simulink model "TCS_Implementation_Controllers"  (R2023b)
settings: Solver=FixedStepDiscrete  StartTime=0.0  StopTime=inf  FixedStep=0.005  RelTol=1e-3  EnableMultiTasking=on
undefined symbols (not defined in the file): bits, DiscIntNeverNeededParam
libraries: stm32f4xxblockslib x19, simulink x17, stm32blockslib x11, dspstat3 x4, embeddedblockslib x3, eeGeneralControl x2, slpidlib x2, mspfiltlib x1
(part 1 of 2)
settings Model: Creator=ADMIN  LastModifiedBy=ADMIN
settings OptimizationCC: EnhancedBackFolding=on  PassReuseOutputArgsAs=Individual arguments  ZeroExternalMemoryAtStartup=off  ZeroInternalMemoryAtStartup=off  MaxStackSize=64  OptimizeBlockOrder=speed  DifferentSizesBufferReuse=on  OptimizationCustomize=off  EfficientTunableParamExpr=on
settings DebuggingCC: MultiTaskDSMMsg=none  TasksWithSamePriorityMsg=none  ParameterPrecisionLossMsg=none  ParameterTunabilityLossMsg=error
settings HardwareCC: ProdBitPerPointer=32  ProdBitPerSizeT=32  ProdBitPerPtrDiffT=32  ProdLargestAtomicInteger=Long  ProdLargestAtomicFloat=Double  ProdWordSize=32  ProdLongLongMode=on  ProdHWDeviceType=ARM Compatible->ARM Cortex
settings SFSimCC: MATLABDynamicMemAlloc=off
settings RTWCC: Description=Embedded Coder  SystemTargetFile=ert.tlc  HardwareBoard=STM32F4xx Based  TemplateMakefile=ert_default_tmf  Toolchain=GNU Tools for ARM Embedded Processors
settings CodeAppCC: ForceParamTrailComments=on  IgnoreCustomStorageClasses=off  OperatorAnnotations=on  SimulinkDataObjDesc=on  SFDataObjDesc=on  InsertBlockDesc=on
settings ERTTargetCC: CodeReplacementLibrary=ARM Cortex-M  ExtModeTransport=3  ExtModeStaticAlloc=on  ExtModeStaticAllocSize=2048  ExtModeMexFile=ext_xcp  ExtModeIntrfLevel=Level2 - Open

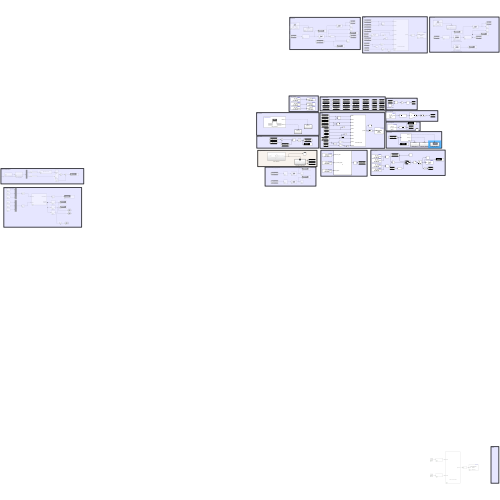
[thumbnail: Simulink's stored preview of the top-level diagram]
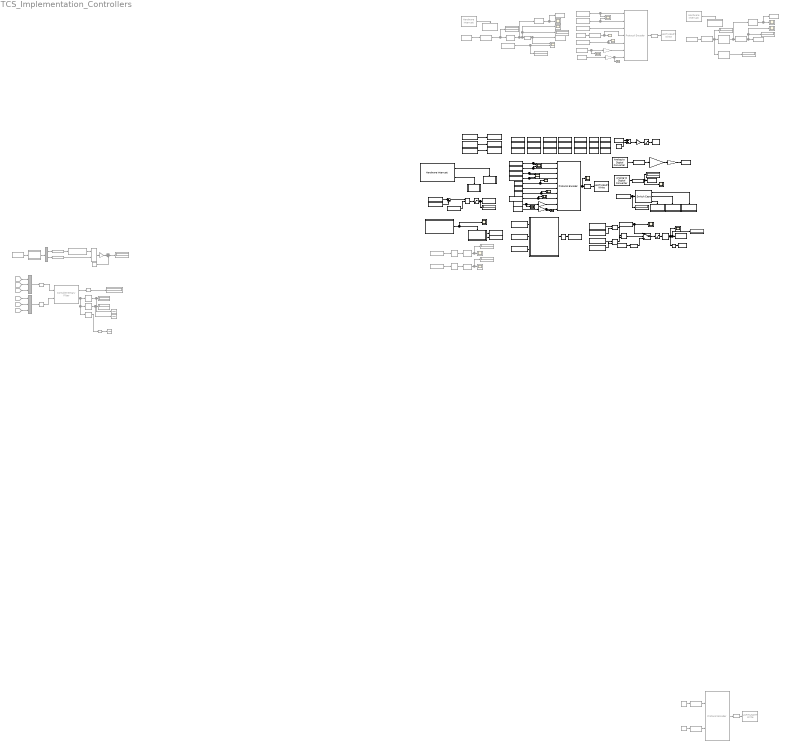
== system TCS_Implementation_Controllers ==
  note: ACC_Calculation_By_System
  note: Torque Sense
  note: Slip_Ratio
  note: WS_Front
  note: Global Variables
  note: Complemetary Filter
  note: WS_Timer
  note: UART
  note: OutPut_DAC
  note: Condition Controller
  note: Controllers
  note: WS_Rear
  note: Throttle Signals
  note: UART
  note: Read Temperature
  note: Signal_LEDs
  note: UART
  note: Current Sense
  note: ACC_Calculation
  AND : Logic  IconShape=distinctive  AllPortsSameDT=off  OutDataTypeStr=boolean
  AND1 : Logic  IconShape=distinctive  AllPortsSameDT=off  OutDataTypeStr=boolean
  Analog to Digital Converter : stm32f4xxblockslib/Analog to Digital Converter  ADCModule=ADC2  ConversionGroup=Regular  TriggerMode=Trigger and read  NumberOfConversions=1  EnableBufferConv=off  BufferLength=1  OutputStatus=off  SampleTime=-1  EnableSimPort=off
  Analog to Digital Converter1 : stm32f4xxblockslib/Analog to Digital Converter  ADCModule=ADC1  ConversionGroup=Regular  TriggerMode=Trigger and read  NumberOfConversions=1  EnableBufferConv=off  BufferLength=1  OutputStatus=off  SampleTime=-1  EnableSimPort=off
  Bitwise Operator7 : simulink/Logic and Bit Operations/Bitwise Operator  Commented=on  logicop=OR  UseBitMask=off  NumInputPorts=2  BitMask=bin2dec('11011001')  BitMaskRealWorld=Stored Integer
  Calculate Acceleration : Subsystem
  Calibrated value : Constant  Value=5  OutDataTypeStr=single
  Complementary Filter : mspfiltlib/Complementary Filter  Commented=on  DispRefFrame=ENU  OrientationFormat=quaternion  AccelerometerGain=0.05  HasMagnetometer=off  MagnetometerGain=0.01  SimulateUsing=Interpreted execution
  Configuration for Accelerometer1 : Constant  Commented=on  Value=hex2dec('0')  OutDataTypeStr=uint8
  Constant1 : Constant  Commented=on  Value=36.35
  Data Store Memory : DataStoreMemory  DataStoreName=WS1_Pulse  WriteAfterWriteMsg=warning  ShowAdditionalParam=off  OutDataTypeStr=uint32
  Data Store Memory1 : DataStoreMemory  DataStoreName=WS2_Pulse  WriteAfterWriteMsg=warning  ShowAdditionalParam=off  OutDataTypeStr=uint32
  Data Store Memory10 : DataStoreMemory  DataStoreName=WS1_ACC_Timer  WriteAfterWriteMsg=warning  ShowAdditionalParam=off  OutDataTypeStr=single
  Data Store Memory11 : DataStoreMemory  DataStoreName=WS2_ACC_Timer  WriteAfterWriteMsg=warning  ShowAdditionalParam=off  OutDataTypeStr=single
  Data Store Memory12 : DataStoreMemory  DataStoreName=WS1_Speed_Timer  WriteAfterWriteMsg=warning  ShowAdditionalParam=off  OutDataTypeStr=single
  Data Store Memory13 : DataStoreMemory  DataStoreName=WS2_Speed_Timer  WriteAfterWriteMsg=warning  ShowAdditionalParam=off  OutDataTypeStr=single
  Data Store Memory14 : DataStoreMemory  DataStoreName=Slip_Ratio  WriteAfterWriteMsg=warning  ShowAdditionalParam=off  OutDataTypeStr=single
  Data Store Memory15 : DataStoreMemory  DataStoreName=DAC_Out  WriteAfterWriteMsg=warning  InitialValue=900  ShowAdditionalParam=off  OutDataTypeStr=uint16
  Data Store Memory16 : DataStoreMemory  DataStoreName=Controller_State  WriteAfterWriteMsg=warning  InitialValue=1100  ShowAdditionalParam=off  OutDataTypeStr=uint16
  Data Store Memory17 : DataStoreMemory  DataStoreName=Roll_Angle  WriteAfterWriteMsg=warning  ShowAdditionalParam=off  OutDataTypeStr=single
  Data Store Memory18 : DataStoreMemory  DataStoreName=Pitch_Angle  WriteAfterWriteMsg=warning  ShowAdditionalParam=off  OutDataTypeStr=single
  Data Store Memory19 : DataStoreMemory  DataStoreName=Yaw_Angle  WriteAfterWriteMsg=warning  ShowAdditionalParam=off  OutDataTypeStr=single
  Data Store Memory2 : DataStoreMemory  DataStoreName=WS1_Speed  WriteAfterWriteMsg=warning  ShowAdditionalParam=off  OutDataTypeStr=single
  Data Store Memory20 : DataStoreMemory  DataStoreName=Yaw_Rate  WriteAfterWriteMsg=warning  ShowAdditionalParam=off  OutDataTypeStr=single
  Data Store Memory3 : DataStoreMemory  DataStoreName=WS2_Speed  WriteAfterWriteMsg=warning  ShowAdditionalParam=off  OutDataTypeStr=single
  Data Store Memory4 : DataStoreMemory  DataStoreName=Throttle_In  WriteAfterWriteMsg=warning  ShowAdditionalParam=off  OutDataTypeStr=single
  Data Store Memory5 : DataStoreMemory  DataStoreName=Current  WriteAfterWriteMsg=warning  ShowAdditionalParam=off  OutDataTypeStr=single
  Data Store Memory6 : DataStoreMemory  DataStoreName=Throttle_Out  WriteAfterWriteMsg=warning  ShowAdditionalParam=off  OutDataTypeStr=single
  Data Store Memory7 : DataStoreMemory  DataStoreName=Torque  WriteAfterWriteMsg=warning  ShowAdditionalParam=off  OutDataTypeStr=single
  Data Store Memory8 : DataStoreMemory  DataStoreName=WS1_ACC  WriteAfterWriteMsg=warning  ShowAdditionalParam=off  OutDataTypeStr=single
  Data Store Memory9 : DataStoreMemory  DataStoreName=WS2_ACC  WriteAfterWriteMsg=warning  ShowAdditionalParam=off  OutDataTypeStr=single
  Data Store Read : DataStoreRead  Commented=on  DataStoreName=WS2_Pulse  IndexOptions=Index vector (dialog)  Indices=1  OutputSizes=1
  Data Store Read1 : DataStoreRead  DataStoreName=WS1_ACC_Timer  IndexOptions=Index vector (dialog)  Indices=1  OutputSizes=1
  Data Store Read10 : DataStoreRead  Commented=on  DataStoreName=WS2_Speed_Timer  IndexOptions=Index vector (dialog)  Indices=1  OutputSizes=1
  Data Store Read11 : DataStoreRead  DataStoreName=WS2_Speed_Timer  IndexOptions=Index vector (dialog)  Indices=1  OutputSizes=1
  Data Store Read12 : DataStoreRead  DataStoreName=Slip_Ratio  IndexOptions=Index vector (dialog)  Indices=1  OutputSizes=1
  Data Store Read13 : DataStoreRead  DataStoreName=Throttle_In  IndexOptions=Index vector (dialog)  Indices=1  OutputSizes=1
  Data Store Read14 : DataStoreRead  DataStoreName=Controller_State  IndexOptions=Index vector (dialog)  Indices=1  OutputSizes=1
  Data Store Read15 : DataStoreRead  DataStoreName=DAC_Out  IndexOptions=Index vector (dialog)  Indices=1  OutputSizes=1
  Data Store Read16 : DataStoreRead  DataStoreName=Current  IndexOptions=Index vector (dialog)  Indices=1  OutputSizes=1
  Data Store Read17 : DataStoreRead  Commented=on  DataStoreName=Slip_Ratio  IndexOptions=Index vector (dialog)  Indices=1  OutputSizes=1
  Data Store Read18 : DataStoreRead  DataStoreName=WS2_ACC_Timer  IndexOptions=Index vector (dialog)  Indices=1  OutputSizes=1
  Data Store Read19 : DataStoreRead  DataStoreName=Torque  IndexOptions=Index vector (dialog)  Indices=1  OutputSizes=1
  Data Store Read2 : DataStoreRead  DataStoreName=WS1_Speed_Timer  IndexOptions=Index vector (dialog)  Indices=1  OutputSizes=1
  Data Store Read20 : DataStoreRead  DataStoreName=Current  IndexOptions=Index vector (dialog)  Indices=1  OutputSizes=1
  Data Store Read22 : DataStoreRead  DataStoreName=Throttle_In  IndexOptions=Index vector (dialog)  Indices=1  OutputSizes=1
  Data Store Read23 : DataStoreRead  Commented=on  DataStoreName=Throttle_In  IndexOptions=Index vector (dialog)  Indices=1  OutputSizes=1
  Data Store Read24 : DataStoreRead  Commented=on  DataStoreName=Current  IndexOptions=Index vector (dialog)  Indices=1  OutputSizes=1
  Data Store Read25 : DataStoreRead  Commented=on  DataStoreName=WS2_ACC_Timer  IndexOptions=Index vector (dialog)  Indices=1  OutputSizes=1
  Data Store Read26 : DataStoreRead  Commented=on  DataStoreName=WS1_Speed_Timer  IndexOptions=Index vector (dialog)  Indices=1  OutputSizes=1
  Data Store Read27 : DataStoreRead  Commented=on  DataStoreName=WS1_Speed_Timer  IndexOptions=Index vector (dialog)  Indices=1  OutputSizes=1
  Data Store Read28 : DataStoreRead  Commented=on  DataStoreName=WS2_Speed_Timer  IndexOptions=Index vector (dialog)  Indices=1  OutputSizes=1
  Data Store Read29 : DataStoreRead  Commented=on  DataStoreName=WS2_Speed_Timer  IndexOptions=Index vector (dialog)  Indices=1  OutputSizes=1
  Data Store Read3 : DataStoreRead  DataStoreName=WS2_Speed_Timer  IndexOptions=Index vector (dialog)  Indices=1  OutputSizes=1
  Data Store Read31 : DataStoreRead  Commented=on  DataStoreName=Throttle_Out  IndexOptions=Index vector (dialog)  Indices=1  OutputSizes=1
  Data Store Read5 : DataStoreRead  DataStoreName=WS1_Speed_Timer  IndexOptions=Index vector (dialog)  Indices=1  OutputSizes=1
  Data Store Read6 : DataStoreRead  DataStoreName=Torque  IndexOptions=Index vector (dialog)  Indices=1  OutputSizes=1
  Data Store Read7 : DataStoreRead  DataStoreName=Throttle_Out  IndexOptions=Index vector (dialog)  Indices=1  OutputSizes=1
  Data Store Read8 : DataStoreRead  Commented=on  DataStoreName=WS1_Pulse  IndexOptions=Index vector (dialog)  Indices=1  OutputSizes=1
  Data Store Read9 : DataStoreRead  DataStoreName=WS2_Speed_Timer  IndexOptions=Index vector (dialog)  Indices=1  OutputSizes=1
  Data Store Write : DataStoreWrite  DataStoreName=Throttle_In  IndexOptions=Index vector (dialog)  Indices=1  OutputSizes=1
  Data Store Write1 : DataStoreWrite  Commented=on  DataStoreName=WS2_Speed  IndexOptions=Index vector (dialog)  Indices=1  OutputSizes=1
  Data Store Write10 : DataStoreWrite  DataStoreName=Slip_Ratio  IndexOptions=Index vector (dialog)  Indices=1  OutputSizes=1
  Data Store Write11 : DataStoreWrite  DataStoreName=Controller_State  IndexOptions=Index vector (dialog)  Indices=1  OutputSizes=1
  Data Store Write15 : DataStoreWrite  DataStoreName=Torque  IndexOptions=Index vector (dialog)  Indices=1  OutputSizes=1
  Data Store Write2 : DataStoreWrite  DataStoreName=Throttle_Out  IndexOptions=Index vector (dialog)  Indices=1  OutputSizes=1
  Data Store Write3 : DataStoreWrite  DataStoreName=Current  IndexOptions=Index vector (dialog)  Indices=1  OutputSizes=1
  Data Store Write4 : DataStoreWrite  DataStoreName=WS1_ACC_Timer  IndexOptions=Index vector (dialog)  Indices=1  OutputSizes=1
  Data Store Write5 : DataStoreWrite  DataStoreName=WS2_ACC_Timer  IndexOptions=Index vector (dialog)  Indices=1  OutputSizes=1
  Data Store Write6 : DataStoreWrite  Commented=on  DataStoreName=WS2_ACC  IndexOptions=Index vector (dialog)  Indices=1  OutputSizes=1
  Data Store Write7 : DataStoreWrite  Commented=on  DataStoreName=WS1_Speed  IndexOptions=Index vector (dialog)  Indices=1  OutputSizes=1
  Data Store Write8 : DataStoreWrite  Commented=on  DataStoreName=WS1_ACC  IndexOptions=Index vector (dialog)  Indices=1  OutputSizes=1
  Data Type Conversion : DataTypeConversion  Commented=on  OutDataTypeStr=double  SaturateOnIntegerOverflow=off  RndMeth=Floor
  Data Type Conversion1 : DataTypeConversion  OutDataTypeStr=single  SaturateOnIntegerOverflow=off  RndMeth=Floor
  Data Type Conversion10 : DataTypeConversion  OutDataTypeStr=uint16  SaturateOnIntegerOverflow=off  RndMeth=Floor
  Data Type Conversion18 : DataTypeConversion  Commented=on  OutDataTypeStr=int16  SaturateOnIntegerOverflow=off  RndMeth=Floor
  Data Type Conversion19 : DataTypeConversion  Commented=on  OutDataTypeStr=int16  SaturateOnIntegerOverflow=off  RndMeth=Floor
  Data Type Conversion{2..3,6,8} (4 alike) : DataTypeConversion  Commented=on  OutDataTypeStr=single  SaturateOnIntegerOverflow=off  RndMeth=Floor
  Data Type Conversion25 : DataTypeConversion  OutDataTypeStr=single  SaturateOnIntegerOverflow=off  RndMeth=Floor
  Data Type Conversion4 : DataTypeConversion  OutDataTypeStr=single  SaturateOnIntegerOverflow=off  RndMeth=Floor
  Data Type Conversion5 : DataTypeConversion  Commented=on  OutDataTypeStr=double  SaturateOnIntegerOverflow=off  RndMeth=Floor
  Data Type Conversion7 : DataTypeConversion  OutDataTypeStr=uint16  SaturateOnIntegerOverflow=off  RndMeth=Floor
  Demux1 : Demux  Commented=on  Outputs=2
  Digital Port Read{1,4..5,10} (4 alike) : stm32f4xxblockslib/Digital Port Read  PortName=GPIOC  PinNumber=[7]  ReadOperation=on  IOAsArray=on  SampleTime=-1  EnableSimPort=off
  Digital Port Read11 : stm32f4xxblockslib/Digital Port Read  PortName=GPIOA  PinNumber=[12]  ReadOperation=on  IOAsArray=on  SampleTime=-1  EnableSimPort=off
  Digital Port Read2 : stm32f4xxblockslib/Digital Port Read  PortName=GPIOA  PinNumber=[11]  ReadOperation=on  IOAsArray=on  SampleTime=-1  EnableSimPort=off
  Digital Port Read6 : stm32f4xxblockslib/Digital Port Read  PortName=GPIOA  PinNumber=[12]  ReadOperation=on  IOAsArray=on  SampleTime=-1  EnableSimPort=off
  Digital Port Read7 : stm32f4xxblockslib/Digital Port Read  PortName=GPIOA  PinNumber=[11]  ReadOperation=on  IOAsArray=on  SampleTime=-1  EnableSimPort=off
  Digital Port Read8 : stm32f4xxblockslib/Digital Port Read  PortName=GPIOA  PinNumber=[12]  ReadOperation=on  IOAsArray=on  SampleTime=-1  EnableSimPort=off
  Digital Port Read9 : stm32f4xxblockslib/Digital Port Read  PortName=GPIOA  PinNumber=[11]  ReadOperation=on  IOAsArray=on  SampleTime=-1  EnableSimPort=off
  Digital Port Write3 : stm32f4xxblockslib/Digital Port Write  PortName=GPIOC  PinNumber=[6]  ReadOperation=off  IOAsArray=on  EnableSimPort=off
  Digital Port Write4 : stm32f4xxblockslib/Digital Port Write  PortName=GPIOC  PinNumber=[8]  ReadOperation=off  IOAsArray=on  EnableSimPort=off
  Digital Port Write5 : stm32f4xxblockslib/Digital Port Write  PortName=GPIOC  PinNumber=[5]  ReadOperation=off  IOAsArray=on  EnableSimPort=off
  Digital to Analog Converter1 : stm32blockslib/Digital to Analog Converter  DACModule=DAC1  TriggerType=Write only  ChannelGroup=Channel1  waveGenEnable=off  waveType=Noise/Triangular  TriggerEnable=on  stepTriggerEnable=on  resetTriggerEnable=on  TrigConfig=Independent trigger  DataLength=12 bits  DataAlignment=Right alignment  dacEnable=off  OutputStatus=off
      settings: LibrarySourceBlock=stm32f4xxblockslib/Digital to Analog Converter
  Discrete Derivative : simulink/Discrete/Discrete Derivative  Commented=on  gainval=(pi*0.41/50)  ICPrevScaledInput=0.0  OutMin=[]  OutMax=[]  OutDataType=fixdt(1, 16)  OutScaling=2^-10  DoSatur=off
  Discrete Derivative2 : simulink/Discrete/Discrete Derivative  Commented=on  gainval=1  ICPrevScaledInput=0  OutMin=[]  OutMax=[]  OutDataTypeStr=single  OutputDataTypeScalingMode=single  OutDataType=fixdt(1, 16)  OutScaling=2^-10  DoSatur=off
  Discrete Derivative3 : simulink/Discrete/Discrete Derivative  Commented=on  gainval=1  ICPrevScaledInput=0  OutMin=[]  OutMax=[]  OutDataTypeStr=single  OutputDataTypeScalingMode=single  OutDataType=fixdt(1, 16)  OutScaling=2^-10  DoSatur=off
  Discrete Derivative5 : simulink/Discrete/Discrete Derivative  Commented=on  gainval=1  ICPrevScaledInput=0.0  OutMin=[]  OutMax=[]  OutDataType=fixdt(1, 16)  OutScaling=2^-10  DoSatur=off
  Discrete Derivative6 : simulink/Discrete/Discrete Derivative  Commented=on  gainval=1  ICPrevScaledInput=0.0  OutMin=[]  OutMax=[]  OutDataType=fixdt(1, 16)  OutScaling=2^-10  DoSatur=off
  Discrete-Time Integrator4 : DiscreteIntegrator  Commented=on  SampleTime=0.005  ICPrevOutput=DiscIntNeverNeededParam  ICPrevScaledInput=DiscIntNeverNeededParam
  Discrete-Time Integrator5 : DiscreteIntegrator  Commented=on  SampleTime=0.005  ICPrevOutput=DiscIntNeverNeededParam  ICPrevScaledInput=DiscIntNeverNeededParam
  Discrete-Time Integrator6 : DiscreteIntegrator  Commented=on  ICPrevOutput=DiscIntNeverNeededParam  ICPrevScaledInput=DiscIntNeverNeededParam
  Display{,1,5..6,8..12,14,17..18} (12 alike) : Display  Commented=on
  Display{2..4,7} (4 alike) : Display
  Divide1 : Product  Inputs=*/
  Filtered Derivative (Discrete or Continuous)1 : eeGeneralControl/Filtered Derivative (Discrete or Continuous)  Commented=on  K=pi*0.4668/50  T=0.1  B=90  A=0  minRatio=5  init_option=Inherited from block input  x0=0  Ts=-1
      settings: LibrarySourceBlock=|
      | ee_sl_lib/General Control/Filtered Derivative
      | (Discrete or Continuous)
  Filtered Derivative (Discrete or Continuous)2 : eeGeneralControl/Filtered Derivative (Discrete or Continuous)  Commented=on  K=60/50  T=0.1  B=2000  A=0  minRatio=5  init_option=Inherited from block input  x0=0  Ts=-1
      settings: LibrarySourceBlock=|
      | ee_sl_lib/General Control/Filtered Derivative
      | (Discrete or Continuous)
  From10 : From  Commented=on  GotoTag=Gryro_Z
  From11 : From  Commented=on  GotoTag=Gryro_Y
  From12 : From  Commented=on  GotoTag=Gryro_X
  From13 : From  Commented=on  GotoTag=Gryro_Z
  From14 : From  Commented=on  GotoTag=Acc_Y
  From15 : From  Commented=on  GotoTag=Acc_X
  Function-Call Subsystem : Subsystem  Commented=on  TreatAsAtomicUnit=on
  Function-Call Subsystem1 : Subsystem  Commented=on  TreatAsAtomicUnit=on
  Function-Call Subsystem2 : Subsystem  TreatAsAtomicUnit=on
  Function-Call Subsystem3 : Subsystem  TreatAsAtomicUnit=on
  Gain : Gain  Gain=(3300/4096)/40  OutDataTypeStr=single
  Gain10 : Gain  Commented=on  Gain=1/340  OutDataTypeStr=single
  Gain11 : Gain  Gain=1.5  OutDataTypeStr=single
  Gain12 : Gain  Commented=on  Gain=3.3/4096  OutDataTypeStr=single
  Gain13 : Gain  Commented=on  Gain=3.3/4096  OutDataTypeStr=single
  Gain2 : Gain  Gain=1/0.75  OutDataTypeStr=single
  Gain3 : Gain  Gain=3.3/4096  OutDataTypeStr=single
  Gain4 : Gain  Gain=3.3/4096  OutDataTypeStr=single
  Get Temp data : Subsystem  Commented=on
  Hardware Interrupt : stm32f4xxblockslib/Hardware Interrupt  Commented=on  ISRGroup=External interrupts (EXTI)  ISRName=EXTI15_10_IRQHandler  ISRNumber=55  EventsList={ 'on', 'EXTI15 Event', '1'; 'off', 'EXTI14 Event', '2'; 'off', 'EXTI13 Event', '3'; 'off', 'EXTI12 Event', '4'; 'off', 'EXTI11 Event', '5'; 'off', 'EXTI10 Event', '6'; 'off', 'Custom event', '7' }  SelectedEvents={'EXTI15 Event'}  TaskPriority=30  DisablePreemption=off  ClearInterruptFlagsAtEndOfEvent=off  InterruptDefinitionFile=$(TARGET_ROOT)/registry/interrupts/STM32F4xxBased_interrupts.xml  HardwareBoard=STM32F4xx Based  EnableSimPort=off
  Hardware Interrupt1 : stm32f4xxblockslib/Hardware Interrupt  Commented=on  ISRGroup=External interrupts (EXTI)  ISRName=EXTI4_IRQHandler  ISRNumber=25  EventsList={ 'on', 'EXTI4 Event', '1'; 'off', 'Custom event', '2' }  SelectedEvents={'EXTI4 Event'}  TaskPriority=30  DisablePreemption=off  ClearInterruptFlagsAtEndOfEvent=off  InterruptDefinitionFile=$(TARGET_ROOT)/registry/interrupts/STM32F4xxBased_interrupts.xml  HardwareBoard=STM32F4xx Based  EnableSimPort=off
  Hardware Interrupt2 : stm32f4xxblockslib/Hardware Interrupt  ISRGroup=Timer (TIM)  ISRName=TIM2_IRQHandler  ISRNumber=43  EventsList={ 'off', 'TIM2 Update', '1'; 'on', 'TIM2 CC1', '2'; 'off', 'TIM2 CC2', '3'; 'on', 'TIM2 CC3', '4'; 'off', 'TIM2 CC4', '5'; 'off', 'TIM2 Trigger', '6'; 'off', 'Custom event', '7' }  SelectedEvents={'TIM2 CC1','TIM2 CC3'}  TaskPriority=5  DisablePreemption=on  ClearInterruptFlagsAtEndOfEvent=on  InterruptDefinitionFile=$(TARGET_ROOT)/registry/interrupts/STM32F4xxBased_interrupts.xml  HardwareBoard=STM32F4xx Based  EnableSimPort=off
  MATLAB Function : MATLAB Function  TreatAsAtomicUnit=on
  Max_Speed : Subsystem
  Median Filter3 : dspstat3/Median Filter  Commented=on  WindowLength=5  SimulateUsing=Interpreted execution
      settings: LibrarySourceBlock=|
      | dspfdesign/Median
      | Filter
  Mux1 : Mux  Commented=on  Inputs=3
  Mux2 : Mux  Commented=on  Inputs=3
  ON_OFF_ACC : Subsystem
  ON_OFF_SlipRatio : Subsystem
  OR : Logic  Operator=OR  IconShape=distinctive  AllPortsSameDT=off  OutDataTypeStr=boolean
  Protocol Encoder1 : embeddedblockslib/Protocol Encoder  Header=0xAA  FieldTable={ 'Field1', '1', 'single', 'Little endian'; 'Field2', '1', 'single', 'Little endian'; 'Field3', '1', 'single', 'Little endian'; 'Field4', '1', 'single', 'Little endian'; 'Field5', '1', 'single', 'Little endian'; 'Field6', '1', 'single', 'Little endian'; 'Field7', '1', 'single', 'Little endian'; 'Field8', '1', 'single', 'Little endian'; 'Field9', '1', 'single', 'Little endian'; 'Field10', '1', 'single', 'Little endian' }  IsChecksumRequired=off  ChecksumAlgorithm=XOR of bytes  ChecksumSize=[]  TerminatorOption=Custom terminator  CustomTerminatorVal=0xCC
      settings: LibrarySourceBlock=stmutilitieslib/Protocol Encoder
  Protocol Encoder2 : embeddedblockslib/Protocol Encoder  Commented=on  Header=0xAA  FieldTable={ 'Field1', '1', 'single', 'Little endian'; 'Field2', '1', 'single', 'Little endian'; 'Field3', '1', 'single', 'Little endian'; 'Field4', '1', 'single', 'Little endian'; 'Field5', '1', 'single', 'Little endian'; 'Field6', '1', 'single', 'Little endian'; 'Field7', '1', 'single', 'Little endian' }  IsChecksumRequired=off  ChecksumAlgorithm=XOR of bytes  ChecksumSize=[]  TerminatorOption=Custom terminator  CustomTerminatorVal=0xCC
      settings: LibrarySourceBlock=stmutilitieslib/Protocol Encoder
  Protocol Encoder3 : embeddedblockslib/Protocol Encoder  Commented=on  Header=0xAA  FieldTable={ 'Field1', '1', 'single', 'Little endian'; 'Field2', '1', 'single', 'Little endian' }  IsChecksumRequired=off  ChecksumAlgorithm=XOR of bytes  ChecksumSize=[]  TerminatorOption=Custom terminator  CustomTerminatorVal=0xCC
      settings: LibrarySourceBlock=stmutilitieslib/Protocol Encoder
  RT : RateTransition  Commented=on  OutPortSampleTime=1
  Random Number : RandomNumber  Commented=on  SampleTime=0.1
  Random Number1 : RandomNumber  Commented=on  SampleTime=0.1
  Rate Transition : RateTransition  OutPortSampleTimeMultiple=2  OutPortSampleTime=0.005
  Rate Transition1 : RateTransition  OutPortSampleTime=0.01
  Rate Transition2 : RateTransition  Commented=on  OutPortSampleTimeMultiple=2  OutPortSampleTime=0.005
  Rate Transition3 : RateTransition  Commented=on  OutPortSampleTimeMultiple=2  OutPortSampleTime=0.005
  Rate Transition4 : RateTransition  Commented=on  OutPortSampleTimeMultiple=6000  OutPortSampleTime=0.01
  Rate Transition5 : RateTransition  Commented=on  OutPortSampleTimeMultiple=6000  OutPortSampleTime=0.03
  Reshape : Reshape  Commented=on  OutputDimensionality=Customize  OutputDimensions=[1,3]
  Reshape1 : Reshape  Commented=on  OutputDimensionality=Customize  OutputDimensions=[1,3]
  Reshape2 : Reshape  Commented=on  OutputDimensions=[1,3]
  Saturation : Saturate  UpperLimit=1.5  LowerLimit=-1.5  OutDataTypeStr=single
  Saturation2 : Saturate  UpperLimit=4095  LowerLimit=860
  Saturation3 : Saturate  UpperLimit=200  LowerLimit=0
  Scope{,2..4,6,8,11..12,24,26} (10 alike) : Scope  Commented=on
  Scope1 : Scope  NumInputPorts=2
  Scope{9..10,14..19,22,25} (10 alike) : Scope
  Scope20 : Scope  Commented=on  NumInputPorts=2
  Scope5 : Scope  NumInputPorts=2
  Scope7 : Scope  Commented=on  NumInputPorts=2
  Selector : Selector  Commented=on  NumberOfDimensions=2  IndexMode=Zero-based  InputPortWidth=3  IndexOptions=Select all,Index vector (dialog)  Indices=0,0  OutputSizes=1,1
  Selector1 : Selector  Commented=on  NumberOfDimensions=2  IndexMode=Zero-based  InputPortWidth=3  IndexOptions=Select all,Index vector (dialog)  Indices=0,1  OutputSizes=1,1
  Selector2 : Selector  Commented=on  NumberOfDimensions=2  IndexMode=Zero-based  InputPortWidth=3  IndexOptions=Select all,Index vector (dialog)  Indices=0,2  OutputSizes=1,1
  Shift Arithmetic7 : ArithShift  Commented=on  BitShiftNumber=8  BitShiftDirection=Left
  Subtract : Sum  Inputs=+-
  Sum : Sum  Inputs=|+-
  Sum1 : Sum  Commented=on  Inputs=|++
  Switch Case : SwitchCase  CaseConditions={1,2}
  Switch1 : Switch  Criteria=u2 > Threshold  SaturateOnIntegerOverflow=off  InputSameDT=off
  Timer Counter : Subsystem
  UART/USART Write1 : stm32blockslib/UART//USART Write  Priority=1  UARTModule=USART3  LengthOfDataToSend=off  BlockingMode=on  BlockingTimeout=0.004  OutputStatus=off
      settings: LibrarySourceBlock=stm32f4xxblockslib/UART//USART Write
  UART/USART Write2 : stm32blockslib/UART//USART Write  Priority=1  Commented=on  UARTModule=USART3  LengthOfDataToSend=off  BlockingMode=off  BlockingTimeout=0.1  OutputStatus=off
      settings: LibrarySourceBlock=stm32f4xxblockslib/UART//USART Write
  UART/USART Write3 : stm32blockslib/UART//USART Write  Priority=1  Commented=on  UARTModule=USART3  LengthOfDataToSend=off  BlockingMode=off  BlockingTimeout=0.1  OutputStatus=off
      settings: LibrarySourceBlock=stm32f4xxblockslib/UART//USART Write
  wires:
  Data Store Read25/1 -> Protocol Encoder2/3
  Data Store Read27/1 -> Protocol Encoder2/1, Scope20/1
  Data Type Conversion25/1 -> Data Store Write2/1
  Protocol Encoder2/1 -> Rate Transition2/1
  Mux1/1 -> Reshape1/1
  Switch Case/3 -> Max_Speed/Action
  Demux1/1 -> Data Type Conversion19/1
  Data Store Read17/1 -> Protocol Encoder2/5, Scope8/1
  Median Filter3/1 -> Protocol Encoder2/4, Scope6/1
  Data Store Read31/1 -> Gain13/1
  Gain12/1 -> Protocol Encoder2/6
  Reshape1/1 -> Complementary Filter/2
  Data Store Read23/1 -> Scope12/1, Gain12/1
  Selector/1 -> Discrete-Time Integrator5/1, Display17/1
  Filtered Derivative (Discrete or Continuous)1/1 -> Discrete Derivative3/1, Data Type Conversion6/1
  RT/1 -> Discrete-Time Integrator6/1
  Gain13/1 -> Scope11/1, Protocol Encoder2/7
  Gain/1 -> Gain2/1
  Switch1/1 -> Saturation2/1
  Hardware Interrupt2/2 -> Function-Call Subsystem3/Trigger
  Selector2/1 -> RT/1
  Gain11/1 -> Saturation3/1
  Data Store Read/1 -> Data Type Conversion/1
  Data Store Read6/1 -> Protocol Encoder1/6
  Data Type Conversion19/1 -> Shift Arithmetic7/1
  Filtered Derivative (Discrete or Continuous)2/1 -> Display1/1
  OR/1 -> Switch1/2
  Selector1/1 -> Discrete-Time Integrator4/1, Display18/1
  Rate Transition2/1 -> UART/USART Write2/1
  Data Type Conversion/1 -> Discrete Derivative/1, Display/1
  Digital Port Read6/1 -> MATLAB Function/3(Normal_Mode)
  Digital Port Read11/1 -> AND1/2
  AND1/1 -> OR/2
  Rate Transition/1 -> UART/USART Write1/1
  Complementary Filter/2 -> Selector2/1, Selector1/1, Selector/1
  Saturation/1 -> Display3/1, Data Store Write10/1
  From12/1 -> Mux1/1
  Configuration for Accelerometer1/1 -> Get Temp data/1(In1)
  From15/1 -> Mux2/1
  Saturation2/1 -> Rate Transition1/1
  From11/1 -> Mux1/2
  From14/1 -> Mux2/2
  Reshape2/1 -> Display14/1
  Shift Arithmetic7/1 -> Bitwise Operator7/1
  Reshape/1 -> Complementary Filter/1
  Complementary Filter/1 -> Reshape2/1
  Rate Transition1/1 -> Display2/1, Digital to Analog Converter1/1, Data Type Conversion25/1, Scope15/1
  Analog to Digital Converter1/1 -> Data Type Conversion4/1
  Constant1/1 -> Sum1/2
  Data Store Read14/1 -> Display7/1, Switch Case/1
  From10/1 -> Mux1/3
  Data Store Read24/1 -> Median Filter3/1
  Digital Port Read1/1 -> AND/1
  Sum1/1 -> Display11/1
  Data Store Read16/1 -> Scope16/1, Protocol Encoder1/7
  Data Type Conversion7/1 -> Switch1/3
  Hardware Interrupt1/1 -> Function-Call Subsystem1/Trigger
  Discrete Derivative/1 -> Display5/1, Scope/1, Data Type Conversion2/1, Discrete Derivative2/1
  Digital Port Read9/1 -> AND/2
  Data Store Read15/1 -> Scope9/1, Switch1/1
  Data Store Read13/1 -> Scope19/1, Gain3/1
  Bitwise Operator7/1 -> Gain10/1
  Demux1/2 -> Data Type Conversion18/1
  Data Store Read22/1 -> Data Type Conversion7/1
  Digital Port Read10/1 -> AND1/1
  Digital Port Read2/1 -> MATLAB Function/2(ACC_Controller_Mode)
  Data Type Conversion6/1 -> Display9/1, Scope3/1, Data Store Write7/1
  Data Store Read11/1 -> Divide1/2
  Data Store Read3/1 -> Protocol Encoder1/2, Scope5/2
  Data Store Read7/1 -> Gain4/1
  Gain2/1 -> Data Store Write3/1
  From13/1 -> Mux2/3
  Data Store Read12/1 -> Scope17/1, Protocol Encoder1/8
  Digital Port Read7/1 -> Digital Port Write4/1
  Sum/1 -> Divide1/1
  Data Type Conversion18/1 -> Bitwise Operator7/2
  Data Store Read10/1 -> Display6/1, Scope7/2
  Data Type Conversion2/1 -> Scope7/1, Data Store Write1/1
  Data Store Read29/1 -> Scope20/2, Protocol Encoder2/2
  Data Type Conversion5/1 -> Filtered Derivative (Discrete or Continuous)2/1, Filtered Derivative (Discrete or Continuous)1/1, Display8/1
  MATLAB Function/1(y) -> Data Type Conversion10/1
  Gain3/1 -> Protocol Encoder1/9
  Hardware Interrupt/1 -> Function-Call Subsystem/Trigger
  Divide1/1 -> Saturation/1
  Protocol Encoder1/1 -> Scope10/1, Rate Transition/1
  Data Store Read2/1 -> Scope5/1, Protocol Encoder1/1
  Hardware Interrupt2/1 -> Function-Call Subsystem2/Trigger
  Digital Port Read8/1 -> Digital Port Write5/1
  Discrete Derivative2/1 -> Data Store Write6/1, Scope2/1
  Gain4/1 -> Protocol Encoder1/10, Scope18/1
  Data Store Read8/1 -> Data Type Conversion5/1
  AND/1 -> OR/1
  Digital Port Read4/1 -> MATLAB Function/1(MaxSpeed_Mode)
  Gain10/1 -> Sum1/1
  Data Store Read5/1 -> Sum/2
  Analog to Digital Converter/1 -> Data Type Conversion1/1
  Data Store Read9/1 -> Sum/1
  Discrete Derivative3/1 -> Data Store Write8/1, Scope4/1
  Digital Port Read5/1 -> Digital Port Write3/1
  Data Type Conversion1/1 -> Scope25/1, Display4/1, Data Store Write/1
  Data Type Conversion4/1 -> Gain/1
  Data Type Conversion10/1 -> Data Store Write11/1
  Get Temp data/1(Out1) -> Demux1/1
  Mux2/1 -> Reshape/1
  Data Store Read1/1 -> Scope1/1, Protocol Encoder1/3
  Data Store Read18/1 -> Scope1/2, Protocol Encoder1/4
  Protocol Encoder3/1 -> Rate Transition3/1
  Rate Transition3/1 -> UART/USART Write3/1
  Random Number1/1 -> Data Type Conversion8/1
  Random Number/1 -> Data Type Conversion3/1
  Data Type Conversion3/1 -> Protocol Encoder3/1
  Data Type Conversion8/1 -> Protocol Encoder3/2
  Data Store Read19/1 -> Scope14/1, Protocol Encoder1/5
  Calibrated value/1 -> Subtract/2
  Data Store Read20/1 -> Subtract/1
  Subtract/1 -> Gain11/1
  Saturation3/1 -> Data Store Write15/1
  Rate Transition4/1 -> Discrete Derivative5/1
  Data Store Read28/1 -> Rate Transition4/1
  Discrete Derivative5/1 -> Display10/1, Scope24/1
  Rate Transition5/1 -> Discrete Derivative6/1
  Discrete Derivative6/1 -> Display12/1, Scope26/1
  Data Store Read26/1 -> Rate Transition5/1
  Timer Counter/1(Out1) -> Calculate Acceleration/Enable, Scope22/1
  Switch Case/2 -> ON_OFF_SlipRatio/Action
  Switch Case/1 -> ON_OFF_ACC/Action
  Calculate Acceleration/1(Outport) -> Data Store Write4/1
  Calculate Acceleration/2(Outport1) -> Data Store Write5/1

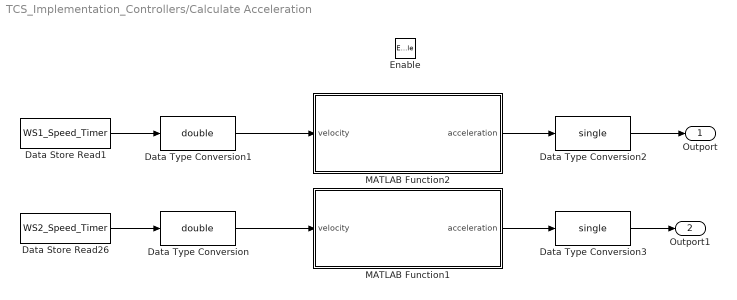
== system TCS_Implementation_Controllers/Calculate Acceleration ==
  Enable : EnablePort
  Data Store Read1 : DataStoreRead  DataStoreName=WS1_Speed_Timer  IndexOptions=Index vector (dialog)  Indices=1  OutputSizes=1
  Data Store Read26 : DataStoreRead  DataStoreName=WS2_Speed_Timer  IndexOptions=Index vector (dialog)  Indices=1  OutputSizes=1
  Data Type Conversion : DataTypeConversion  OutDataTypeStr=double  SaturateOnIntegerOverflow=off  RndMeth=Floor
  Data Type Conversion1 : DataTypeConversion  OutDataTypeStr=double  SaturateOnIntegerOverflow=off  RndMeth=Floor
  Data Type Conversion2 : DataTypeConversion  OutDataTypeStr=single  SaturateOnIntegerOverflow=off  RndMeth=Floor
  Data Type Conversion3 : DataTypeConversion  OutDataTypeStr=single  SaturateOnIntegerOverflow=off  RndMeth=Floor
  MATLAB Function1 : MATLAB Function  TreatAsAtomicUnit=on
  MATLAB Function2 : MATLAB Function  TreatAsAtomicUnit=on
  Outport : Outport
  Outport1 : Outport  Port=2
  wires:
  Data Store Read26/1 -> Data Type Conversion/1
  Data Type Conversion/1 -> MATLAB Function1/1(velocity)
  MATLAB Function1/1(acceleration) -> Data Type Conversion3/1
  Data Type Conversion1/1 -> MATLAB Function2/1(velocity)
  MATLAB Function2/1(acceleration) -> Data Type Conversion2/1
  Data Store Read1/1 -> Data Type Conversion1/1
  Data Type Conversion3/1 -> Outport1/1
  Data Type Conversion2/1 -> Outport/1

== system TCS_Implementation_Controllers/Function-Call Subsystem ==
  function : TriggerPort  TriggerType=function-call  VariantControl=(inherit)
  Constant : Constant
  Data Store Read : DataStoreRead  DataStoreName=WS2_Pulse  IndexOptions=Index vector (dialog)  Indices=1  OutputSizes=1
  Data Store Write : DataStoreWrite  DataStoreName=WS2_Pulse  IndexOptions=Index vector (dialog)  Indices=1  OutputSizes=1
  Sum : Sum  Inputs=|++  OutDataTypeStr=uint32
  wires:
  Sum/1 -> Data Store Write/1
  Constant/1 -> Sum/1
  Data Store Read/1 -> Sum/2

== system TCS_Implementation_Controllers/Function-Call Subsystem1 ==
  function : TriggerPort  TriggerType=function-call  VariantControl=(inherit)
  Constant : Constant
  Data Store Read : DataStoreRead  DataStoreName=WS1_Pulse  IndexOptions=Index vector (dialog)  Indices=1  OutputSizes=1
  Data Store Write : DataStoreWrite  DataStoreName=WS1_Pulse  IndexOptions=Index vector (dialog)  Indices=1  OutputSizes=1
  Sum : Sum  Inputs=|++  OutDataTypeStr=uint32
  wires:
  Sum/1 -> Data Store Write/1
  Constant/1 -> Sum/1
  Data Store Read/1 -> Sum/2

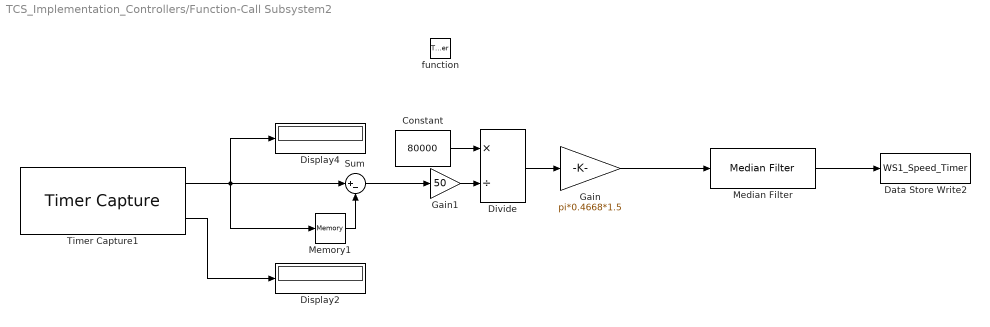
== system TCS_Implementation_Controllers/Function-Call Subsystem2 ==
  function : TriggerPort  TriggerType=function-call  VariantControl=(inherit)
  Constant : Constant  Value=80000
  Data Store Write2 : DataStoreWrite  DataStoreName=WS1_Speed_Timer  IndexOptions=Index vector (dialog)  Indices=1  OutputSizes=1
  Display2 : Display
  Display4 : Display
  Divide : Product  Inputs=*/  OutDataTypeStr=double
  Gain : Gain  Gain=pi*0.4668*1.5  OutDataTypeStr=single
  Gain1 : Gain  Gain=50
  Median Filter : dspstat3/Median Filter  WindowLength=5  SimulateUsing=Interpreted execution
      settings: LibrarySourceBlock=|
      | dspfdesign/Median
      | Filter
  Memory1 : Memory  InheritSampleTime=on  LinearizeMemory=on  LinearizeAsDelay=on
  Sum : Sum  Inputs=|+-  OutDataTypeStr=double
  Timer Capture1 : stm32blockslib/Timer Capture  TimerModule=TIM2  SelectedChannel=CH1  CaptureLength=1  OutputDataLength=off  OutputOverrunStatus=on  OutputDirection=off  SampleTime=-1
      settings: LibrarySourceBlock=stm32f4xxblockslib/Timer Capture
  wires:
  Divide/1 -> Gain/1
  Memory1/1 -> Sum/2
  Timer Capture1/2 -> Display2/1
  Timer Capture1/1 -> Memory1/1, Sum/1, Display4/1
  Sum/1 -> Gain1/1
  Constant/1 -> Divide/1
  Gain/1 -> Median Filter/1
  Gain1/1 -> Divide/2
  Median Filter/1 -> Data Store Write2/1

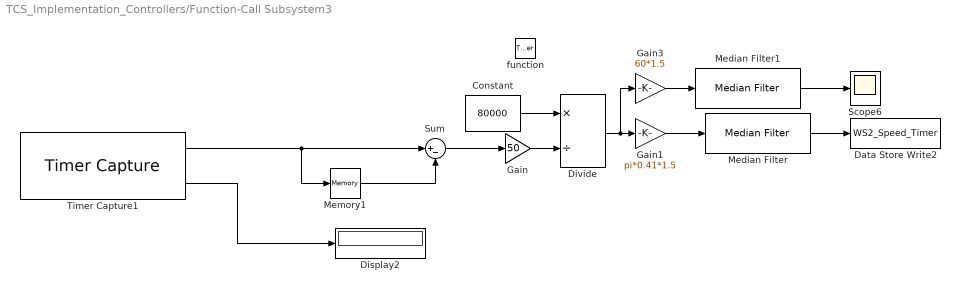
== system TCS_Implementation_Controllers/Function-Call Subsystem3 ==
  function : TriggerPort  TriggerType=function-call  VariantControl=(inherit)
  Constant : Constant  Value=80000
  Data Store Write2 : DataStoreWrite  DataStoreName=WS2_Speed_Timer  IndexOptions=Index vector (dialog)  Indices=1  OutputSizes=1
  Display2 : Display
  Divide : Product  Inputs=*/  OutDataTypeStr=double
  Gain : Gain  Gain=50
  Gain1 : Gain  Gain=pi*0.41*1.5  OutDataTypeStr=single
  Gain3 : Gain  Gain=60*1.5  OutDataTypeStr=single
  Median Filter : dspstat3/Median Filter  WindowLength=5  SimulateUsing=Interpreted execution
      settings: LibrarySourceBlock=|
      | dspfdesign/Median
      | Filter
  Median Filter1 : dspstat3/Median Filter  WindowLength=5  SimulateUsing=Interpreted execution
      settings: LibrarySourceBlock=|
      | dspfdesign/Median
      | Filter
  Memory1 : Memory  InheritSampleTime=on  LinearizeMemory=on  LinearizeAsDelay=on
  Scope6 : Scope
  Sum : Sum  Inputs=|+-  OutDataTypeStr=double
  Timer Capture1 : stm32blockslib/Timer Capture  TimerModule=TIM2  SelectedChannel=CH3  CaptureLength=1  OutputDataLength=off  OutputOverrunStatus=on  OutputDirection=off  SampleTime=-1
      settings: LibrarySourceBlock=stm32f4xxblockslib/Timer Capture
  wires:
  Divide/1 -> Gain3/1, Gain1/1
  Timer Capture1/2 -> Display2/1
  Sum/1 -> Gain/1
  Constant/1 -> Divide/1
  Gain/1 -> Divide/2
  Timer Capture1/1 -> Memory1/1, Sum/1
  Memory1/1 -> Sum/2
  Gain1/1 -> Median Filter/1
  Median Filter/1 -> Data Store Write2/1
  Gain3/1 -> Median Filter1/1
  Median Filter1/1 -> Scope6/1

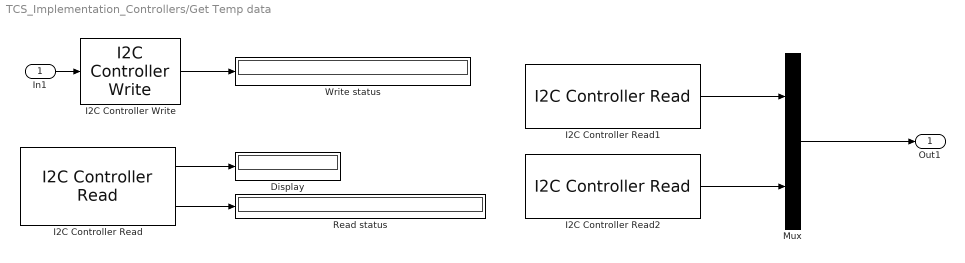
== system TCS_Implementation_Controllers/Get Temp data ==
  In1 : Inport
  Display : Display
      settings: Format=hex (Stored Integer)
  I2C Controller Read : stm32blockslib/I2C Controller Read  I2CModule=I2C1  Mode=Controller  AddressingMode=7-bits  PeripheralByteOrder=BigEndian  OwnPeripheralAddress=uint8(170)  PeripheralAddressVia=Dialog  PeripheralAddress=104  RegisterAddressMode=on  RegisterAddressVia=Dialog  RegisterAddress=107  RepeatedStart=off  NoAck=off  OutputStatus=on  BlockMode=Receive  DataType=uint8  DataLength=1  Timeout=0.001  SampleTime=0.005
      settings: LibrarySourceBlock=stm32f4xxblockslib/I2C Controller Read
  I2C Controller Read1 : stm32blockslib/I2C Controller Read  I2CModule=I2C1  Mode=Controller  AddressingMode=7-bits  PeripheralByteOrder=BigEndian  OwnPeripheralAddress=uint8(170)  PeripheralAddressVia=Dialog  PeripheralAddress=104  RegisterAddressMode=on  RegisterAddressVia=Dialog  RegisterAddress=65  RepeatedStart=off  NoAck=off  OutputStatus=off  BlockMode=Receive  DataType=uint8  DataLength=1  Timeout=0.001  SampleTime=0.005
      settings: LibrarySourceBlock=stm32f4xxblockslib/I2C Controller Read
  I2C Controller Read2 : stm32blockslib/I2C Controller Read  I2CModule=I2C1  Mode=Controller  AddressingMode=7-bits  PeripheralByteOrder=BigEndian  OwnPeripheralAddress=uint8(170)  PeripheralAddressVia=Dialog  PeripheralAddress=104  RegisterAddressMode=on  RegisterAddressVia=Dialog  RegisterAddress=66  RepeatedStart=off  NoAck=off  OutputStatus=off  BlockMode=Receive  DataType=uint8  DataLength=1  Timeout=0.001  SampleTime=0.005
      settings: LibrarySourceBlock=stm32f4xxblockslib/I2C Controller Read
  I2C Controller Write : stm32blockslib/I2C Controller Write  I2CModule=I2C1  Mode=Controller  AddressingMode=7-bits  PeripheralByteOrder=BigEndian  OwnPeripheralAddress=uint8(170)  PeripheralAddressVia=Dialog  PeripheralAddress=104  RegisterAddressMode=on  RegisterAddressVia=Dialog  RegisterAddress=107  RepeatedStart=off  NoAck=off  OutputStatus=on  BlockMode=Transmit  DataType=uint8  DataLength=1  Timeout=0.001  SampleTime=-1
      settings: LibrarySourceBlock=stm32f4xxblockslib/I2C Controller Write
  Mux : Mux  Inputs=2
  Read status : Display
      settings: Format=hex (Stored Integer)
  Write status : Display
      settings: Format=hex (Stored Integer)
  Out1 : Outport  VectorParamsAs1DForOutWhenUnconnected=off
  wires:
  I2C Controller Write/1 -> Write status/1
  In1/1 -> I2C Controller Write/1
  I2C Controller Read1/1 -> Mux/1
  I2C Controller Read2/1 -> Mux/2
  Mux/1 -> Out1/1
  I2C Controller Read/1 -> Display/1
  I2C Controller Read/2 -> Read status/1

== system TCS_Implementation_Controllers/Max_Speed ==
  Action Port : ActionPort  ActionPortLabel=default:
  Compare To Constant : simulink/Logic and Bit Operations/Compare To Constant  relop===  const=0  OutDataTypeStr=boolean
  Digital Port Read3 : stm32f4xxblockslib/Digital Port Read  PortName=GPIOC  PinNumber=[7]  ReadOperation=on  IOAsArray=on  SampleTime=-1  EnableSimPort=off
  Subsystem : Subsystem
  Subsystem1 : Subsystem
  wires:
  Digital Port Read3/1 -> Subsystem/Enable, Compare To Constant/1
  Compare To Constant/1 -> Subsystem1/Enable

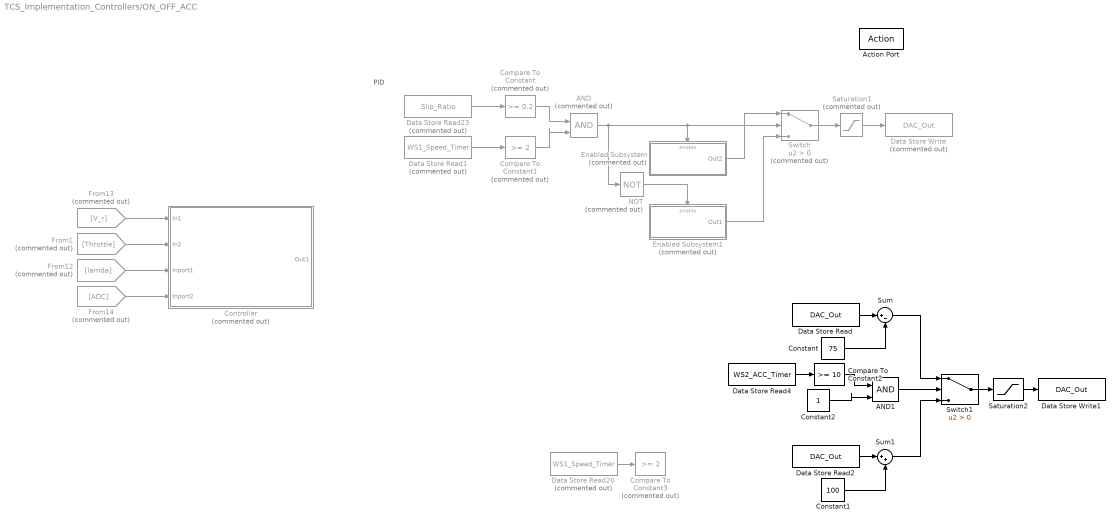
== system TCS_Implementation_Controllers/ON_OFF_ACC ==
  note: PID
  Action Port : ActionPort  ActionPortLabel=case [ 1 ]:
  AND : Logic  Commented=on  IconShape=distinctive  AllPortsSameDT=off  OutDataTypeStr=boolean
  AND1 : Logic  IconShape=distinctive  AllPortsSameDT=off  OutDataTypeStr=boolean
  Compare To Constant : simulink/Logic and Bit Operations/Compare To Constant  Commented=on  relop=>=  const=0.2  OutDataTypeStr=boolean
  Compare To Constant1 : simulink/Logic and Bit Operations/Compare To Constant  Commented=on  relop=>=  const=2  OutDataTypeStr=boolean
  Compare To Constant2 : simulink/Logic and Bit Operations/Compare To Constant  relop=>=  const=10  OutDataTypeStr=boolean
  Compare To Constant3 : simulink/Logic and Bit Operations/Compare To Constant  Commented=on  relop=>=  const=2  OutDataTypeStr=boolean
  Constant : Constant  Value=75  OutDataTypeStr=uint16
  Constant1 : Constant  Value=100  OutDataTypeStr=uint16
  Constant2 : Constant
  "Controller " : Subsystem  Commented=on  TreatAsAtomicUnit=on
  Data Store Read : DataStoreRead  DataStoreName=DAC_Out  IndexOptions=Index vector (dialog)  Indices=1  OutputSizes=1
  Data Store Read1 : DataStoreRead  Commented=on  DataStoreName=WS1_Speed_Timer  IndexOptions=Index vector (dialog)  Indices=1  OutputSizes=1
  Data Store Read2 : DataStoreRead  DataStoreName=DAC_Out  IndexOptions=Index vector (dialog)  Indices=1  OutputSizes=1
  Data Store Read20 : DataStoreRead  Commented=on  DataStoreName=WS1_Speed_Timer  IndexOptions=Index vector (dialog)  Indices=1  OutputSizes=1
  Data Store Read23 : DataStoreRead  Commented=on  DataStoreName=Slip_Ratio  IndexOptions=Index vector (dialog)  Indices=1  OutputSizes=1
  Data Store Read4 : DataStoreRead  DataStoreName=WS2_ACC_Timer  IndexOptions=Index vector (dialog)  Indices=1  OutputSizes=1
  Data Store Write : DataStoreWrite  Commented=on  DataStoreName=DAC_Out  IndexOptions=Index vector (dialog)  Indices=1  OutputSizes=1
  Data Store Write1 : DataStoreWrite  DataStoreName=DAC_Out  IndexOptions=Index vector (dialog)  Indices=1  OutputSizes=1
  Enabled Subsystem : Subsystem  Commented=on  TreatAsAtomicUnit=on
  Enabled Subsystem1 : Subsystem  Commented=on  TreatAsAtomicUnit=on
  From1 : From  Commented=on  GotoTag=Throttle  TagVisibility=global
  From12 : From  Commented=on  GotoTag=lamda  TagVisibility=global
  From13 : From  Commented=on  GotoTag=V_r  TagVisibility=global
  From14 : From  Commented=on  GotoTag=ADC  TagVisibility=global
  NOT : Logic  Commented=on  Operator=NOT  IconShape=distinctive  AllPortsSameDT=off  OutDataTypeStr=boolean
  Saturation1 : Saturate  Commented=on  UpperLimit=4095  LowerLimit=1200  OutDataTypeStr=uint16
  Saturation2 : Saturate  UpperLimit=4095  LowerLimit=990
  Sum : Sum  Inputs=|+-
  Sum1 : Sum  Inputs=|++
  Switch : Switch  Commented=on  Criteria=u2 > Threshold  SaturateOnIntegerOverflow=off  InputSameDT=off
  Switch1 : Switch  Criteria=u2 > Threshold  SaturateOnIntegerOverflow=off  InputSameDT=off
  wires:
  Data Store Read1/1 -> Compare To Constant1/1
  Data Store Read23/1 -> Compare To Constant/1
  Compare To Constant/1 -> AND/1
  Compare To Constant1/1 -> AND/2
  AND/1 -> Switch/2, Enabled Subsystem/Enable, NOT/1
  NOT/1 -> Enabled Subsystem1/Enable
  Switch/1 -> Saturation1/1
  Saturation1/1 -> Data Store Write/1
  Enabled Subsystem1/1(Out1) -> Switch/3
  Enabled Subsystem/1(Out2) -> Switch/1
  AND1/1 -> Switch1/2
  Sum1/1 -> Switch1/3
  Constant/1 -> Sum/2
  Data Store Read4/1 -> Compare To Constant2/1
  Data Store Read2/1 -> Sum1/1
  Sum/1 -> Switch1/1
  Compare To Constant2/1 -> AND1/1
  Data Store Read/1 -> Sum/1
  Switch1/1 -> Saturation2/1
  Saturation2/1 -> Data Store Write1/1
  Data Store Read20/1 -> Compare To Constant3/1
  Constant1/1 -> Sum1/2
  From14/1 -> "Controller "/4(Inport2)
  From13/1 -> "Controller "/1(In1)
  From12/1 -> "Controller "/3(Inport1)
  From1/1 -> "Controller "/2(In2)
  Constant2/1 -> AND1/2

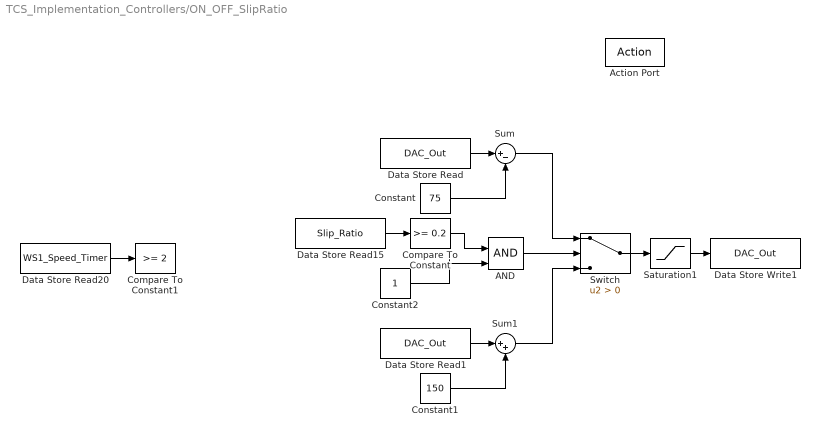
== system TCS_Implementation_Controllers/ON_OFF_SlipRatio ==
  Action Port : ActionPort  ActionPortLabel=case [ 2 ]:
  AND : Logic  IconShape=distinctive  AllPortsSameDT=off  OutDataTypeStr=boolean
  Compare To Constant : simulink/Logic and Bit Operations/Compare To Constant  relop=>=  const=0.2  OutDataTypeStr=boolean
  Compare To Constant1 : simulink/Logic and Bit Operations/Compare To Constant  relop=>=  const=2  OutDataTypeStr=boolean
  Constant : Constant  Value=75  OutDataTypeStr=uint16
  Constant1 : Constant  Value=150  OutDataTypeStr=uint16
  Constant2 : Constant
  Data Store Read : DataStoreRead  DataStoreName=DAC_Out  IndexOptions=Index vector (dialog)  Indices=1  OutputSizes=1
  Data Store Read1 : DataStoreRead  DataStoreName=DAC_Out  IndexOptions=Index vector (dialog)  Indices=1  OutputSizes=1
  Data Store Read15 : DataStoreRead  DataStoreName=Slip_Ratio  IndexOptions=Index vector (dialog)  Indices=1  OutputSizes=1
  Data Store Read20 : DataStoreRead  DataStoreName=WS1_Speed_Timer  IndexOptions=Index vector (dialog)  Indices=1  OutputSizes=1
  Data Store Write1 : DataStoreWrite  DataStoreName=DAC_Out  IndexOptions=Index vector (dialog)  Indices=1  OutputSizes=1
  Saturation1 : Saturate  UpperLimit=4095  LowerLimit=990
  Sum : Sum  Inputs=|+-
  Sum1 : Sum  Inputs=|++
  Switch : Switch  Criteria=u2 > Threshold  SaturateOnIntegerOverflow=off  InputSameDT=off
  wires:
  Data Store Read/1 -> Sum/1
  Constant/1 -> Sum/2
  Data Store Read15/1 -> Compare To Constant/1
  Data Store Read20/1 -> Compare To Constant1/1
  Compare To Constant/1 -> AND/1
  AND/1 -> Switch/2
  Switch/1 -> Saturation1/1
  Saturation1/1 -> Data Store Write1/1
  Sum/1 -> Switch/1
  Constant1/1 -> Sum1/2
  Data Store Read1/1 -> Sum1/1
  Sum1/1 -> Switch/3
  Constant2/1 -> AND/2

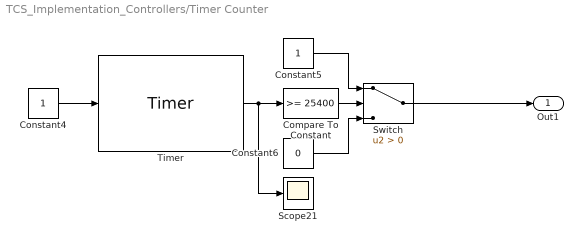
== system TCS_Implementation_Controllers/Timer Counter ==
  Compare To Constant : simulink/Logic and Bit Operations/Compare To Constant  relop=>=  const=25400  OutDataTypeStr=boolean
  Constant4 : Constant
  Constant5 : Constant
  Constant6 : Constant  Value=0
  Scope21 : Scope
  Switch : Switch  Criteria=u2 > Threshold  SaturateOnIntegerOverflow=off  InputSameDT=off
  Timer : stm32blockslib/Timer  Priority=4  TimerModule=TIM5  EnableFrequencyInput=off  EnableCounterInput=on  EnableMainOutputInput=off  SetRCAfterCE=off  OutputDirection=off  OutputMainOutputEnableStatus=off  SampleTime=-1  EnableUpdateEvent=off  EnableCaptureCompare1Event=off  EnableCaptureCompare2Event=off  EnableCaptureCompare3Event=off  EnableCaptureCompare4Event=off  EnableTriggerEvent=off  EnableBreakEvent=off  EnableBreakEvent2=off  EnableCOMGenerationEvent=off  ProcessorFamily=STM32F7
      settings: LibrarySourceBlock=stm32f4xxblockslib/Timer
  Out1 : Outport
  wires:
  Constant5/1 -> Switch/1
  Timer/1 -> Scope21/1, Compare To Constant/1
  Compare To Constant/1 -> Switch/2
  Constant6/1 -> Switch/3
  Constant4/1 -> Timer/1
  Switch/1 -> Out1/1

== system TCS_Implementation_Controllers/Max_Speed/Subsystem ==
  Enable : EnablePort
  Constant : Constant  Value=4095  OutDataTypeStr=uint16
  Data Store Write1 : DataStoreWrite  DataStoreName=DAC_Out  IndexOptions=Index vector (dialog)  Indices=1  OutputSizes=1
  wires:
  Constant/1 -> Data Store Write1/1

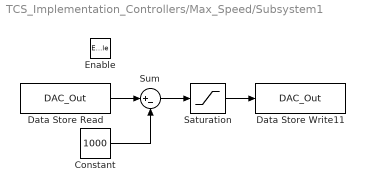
== system TCS_Implementation_Controllers/Max_Speed/Subsystem1 ==
  Enable : EnablePort
  Constant : Constant  Value=1000  OutDataTypeStr=uint16
  Data Store Read : DataStoreRead  DataStoreName=DAC_Out  IndexOptions=Index vector (dialog)  Indices=1  OutputSizes=1
  Data Store Write11 : DataStoreWrite  DataStoreName=DAC_Out  IndexOptions=Index vector (dialog)  Indices=1  OutputSizes=1
  Saturation : Saturate  UpperLimit=4095  LowerLimit=990
  Sum : Sum  Inputs=|+-
  wires:
  Data Store Read/1 -> Sum/1
  Constant/1 -> Sum/2
  Sum/1 -> Saturation/1
  Saturation/1 -> Data Store Write11/1

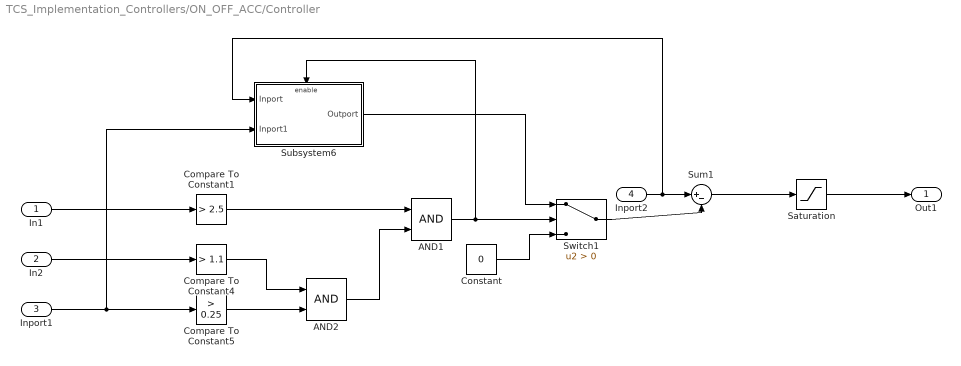
== system TCS_Implementation_Controllers/ON_OFF_ACC/Controller  ==
  In1 : Inport
  In2 : Inport  Port=2
  Inport1 : Inport  Port=3
  Inport2 : Inport  Port=4
  AND1 : Logic  IconShape=distinctive  AllPortsSameDT=off  OutDataTypeStr=boolean
  AND2 : Logic  IconShape=distinctive  AllPortsSameDT=off  OutDataTypeStr=boolean
  Compare To Constant1 : simulink/Logic and Bit Operations/Compare To Constant  relop=>  const=2.5  OutDataTypeStr=boolean
  Compare To Constant4 : simulink/Logic and Bit Operations/Compare To Constant  relop=>  const=1.1  OutDataTypeStr=boolean
  Compare To Constant5 : simulink/Logic and Bit Operations/Compare To Constant  relop=>  const=0.25  OutDataTypeStr=boolean
  Constant : Constant  Value=0
  Saturation : Saturate  UpperLimit=4096  LowerLimit=1000
  Subsystem6 : Subsystem
  Sum1 : Sum  Inputs=|+-
  Switch1 : Switch  Criteria=u2 > Threshold  SaturateOnIntegerOverflow=off  InputSameDT=off
  Out1 : Outport
  wires:
  Compare To Constant5/1 -> AND2/2
  Compare To Constant4/1 -> AND2/1
  In2/1 -> Compare To Constant4/1
  Inport1/1 -> Subsystem6/2(Inport1), Compare To Constant5/1
  In1/1 -> Compare To Constant1/1
  AND2/1 -> AND1/2
  AND1/1 -> Switch1/2, Subsystem6/Enable
  Subsystem6/1(Outport) -> Switch1/1
  Constant/1 -> Switch1/3
  Switch1/1 -> Sum1/2
  Inport2/1 -> Subsystem6/1(Inport), Sum1/1
  Sum1/1 -> Saturation/1
  Saturation/1 -> Out1/1
  Compare To Constant1/1 -> AND1/1
